simulink model "simpleTankTest"  (R2020b)
settings: Solver=VariableStepAuto  StartTime=0.0  StopTime=50  RelTol=1e-3
libraries: fl_lib x11, nesl_utility x10, SimscapeCustomBlocks_lib x2
settings Model: Creator=Edward  LastModifiedBy=Edward

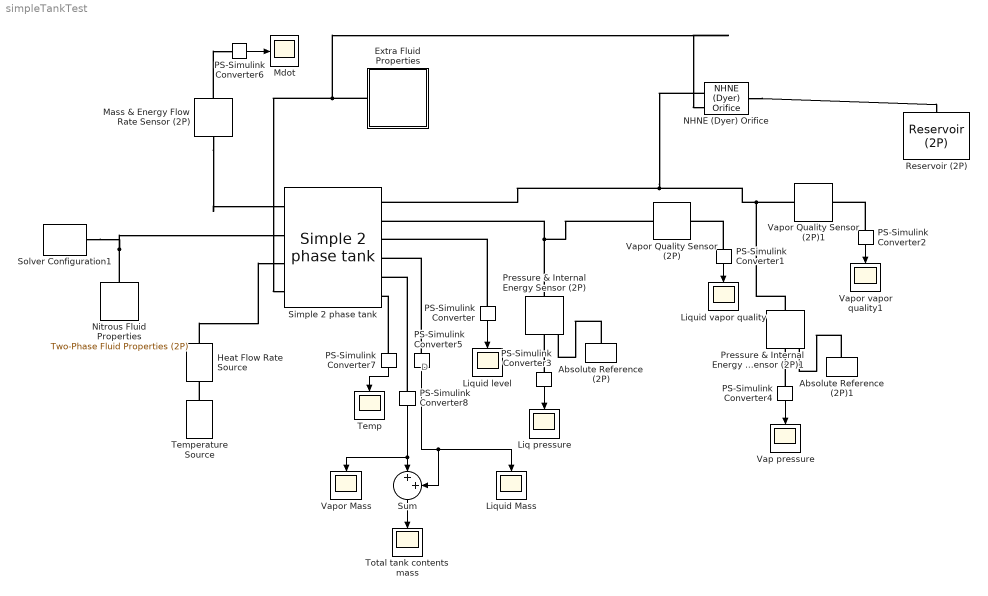
== system simpleTankTest ==
  note: D
  Absolute Reference (2P) : fl_lib/Two-Phase Fluid/Elements/Absolute Reference (2P)
      settings: SourceProductBaseCode=SS
  Absolute Reference (2P)1 : fl_lib/Two-Phase Fluid/Elements/Absolute Reference (2P)
      settings: SourceProductBaseCode=SS
  Extra Fluid Properties : Subsystem  ReferencedSubsystem=nitrousExtraFluidProps
  Heat Flow Rate Source : fl_lib/Thermal/Thermal Sources/Heat Flow Rate Source  heat_flow=900 W
      settings: SourceProductBaseCode=SS  InternalSimscapePortConfiguration="{\"Bottom\":[],\"Left\":[{\"id\":\"B\",\"label\":\"B\",\"type\":\"foundation.thermal.thermal\"}],\"Right\":[{\"id\":\"A\",\"label\":\"A\",\"type\":\"foundation.thermal.thermal\"}],\"Top\":[]}"
  Liq pressure : Scope
  Liquid Mass : Scope
  Liquid level : Scope
  Liquid vapor quality : Scope
  Mass & Energy Flow Rate Sensor (2P) : fl_lib/Two-Phase Fluid/Sensors/Mass & Energy Flow Rate Sensor (2P)
      settings: SourceProductBaseCode=SS  InternalSimscapePortConfiguration="{\"Bottom\":[],\"Left\":[{\"id\":\"A\",\"label\":\"A\",\"type\":\"foundation.two_phase_fluid.two_phase_fluid\"}],\"Right\":[{\"id\":\"B\",\"label\":\"B\",\"type\":\"foundation.two_phase_fluid.two_phase_fluid\"},{\"id\":\"M\",\"label\":\"M\",\"type\":\"output\"},{\"id\":\"PHI\",\"label\":\"Phi\",\"type\":\"output\"}],\"Top\":[]}"
  Mdot : Scope
  NHNE (Dyer) Orifice : SimscapeCustomBlocks_lib/NHNE (Dyer) Orifice  area=0.01 m^2  orifice_area=0.25*pi*(1.5e-3)^2 m^2  Cd=0.8
      settings: InternalSimscapePortConfiguration="{\"Bottom\":[],\"Left\":[{\"id\":\"A\",\"label\":\"A\",\"type\":\"foundation.two_phase_fluid.two_phase_fluid\"}],\"Right\":[{\"id\":\"B\",\"label\":\"B\",\"type\":\"foundation.two_phase_fluid.two_phase_fluid\"}],\"Top\":[{\"id\":\"Props\",\"label\":\"Props\",\"type\":\"SimscapeCustomBlocks.customFluidDomain.extra_two_phase_fluid_props\"}]}"
  Nitrous Fluid Properties : fl_lib/Two-Phase Fluid/Utilities/Two-Phase Fluid Properties (2P)  u_min=Sim.nitrousFluidTable.u_min kJ/kg  u_max=Sim.nitrousFluidTable.u_max kJ/kg  unorm_liq=Sim.nitrousFluidTable.liquid.unorm  unorm_vap=Sim.nitrousFluidTable.vapor.unorm  p_TLU=Sim.nitrousFluidTable.p MPa  v_liq=Sim.nitrousFluidTable.liquid.v m^3/kg  v_vap=Sim.nitrousFluidTable.vapor.v m^3/kg  s_liq=Sim.nitrousFluidTable.liquid.s kJ/kg/K  s_vap=Sim.nitrousFluidTable.vapor.s kJ/kg/K  T_liq=Sim.nitrousFluidTable.liquid.T K  T_vap=Sim.nitrousFluidTable.vapor.T K  nu_liq=Sim.nitrousFluidTable.liquid.nu mm^2/s  nu_vap=Sim.nitrousFluidTable.vapor.nu mm^2/s  k_liq=Sim.nitrousFluidTable.liquid.k W/(m*K)  k_vap=Sim.nitrousFluidTable.vapor.k W/(m*K)  Pr_liq=Sim.nitrousFluidTable.liquid.Pr  Pr_vap=Sim.nitrousFluidTable.vapor.Pr  u_sat_liq=Sim.nitrousFluidTable.liquid.u_sat kJ/kg  u_sat_vap=Sim.nitrousFluidTable.vapor.u_sat kJ/kg  p_crit=Sim.nitrousFluidTable.p_crit MPa  critical_region=foundation.enum.critical_region.clip  p_crit_fraction=0.12  p_atm=0.101325 MPa  q_rev=0.01 Pa
      settings: SourceProductBaseCode=SS  InternalSimscapePortConfiguration="{\"Bottom\":[],\"Left\":[],\"Right\":[{\"id\":\"A\",\"label\":\"\",\"type\":\"foundation.two_phase_fluid.two_phase_fluid\"}],\"Top\":[]}"
  PS-Simulink Converter{,1..8} (9 alike) : nesl_utility/PS-Simulink Converter  PhysicalDomain=network_engine_domain  SubClassName=ps_output  LeftPortType=input  RightPortType=output  PseudoPeriodic=off  Frequencies=[]  Unit=inherit  AffineConversion=off
  Pressure & Internal Energy Sensor (2P) : fl_lib/Two-Phase Fluid/Sensors/Pressure & Internal Energy Sensor (2P)
      settings: SourceProductBaseCode=SS  InternalSimscapePortConfiguration="{\"Bottom\":[],\"Left\":[{\"id\":\"A\",\"label\":\"A\",\"type\":\"foundation.two_phase_fluid.two_phase_fluid\"}],\"Right\":[{\"id\":\"B\",\"label\":\"B\",\"type\":\"foundation.two_phase_fluid.two_phase_fluid\"},{\"id\":\"P\",\"label\":\"P\",\"type\":\"output\"},{\"id\":\"U\",\"label\":\"U\",\"type\":\"output\"}],\"Top\":[]}"
  Pressure & Internal Energy Sensor (2P)1 : fl_lib/Two-Phase Fluid/Sensors/Pressure & Internal Energy Sensor (2P)
      settings: SourceProductBaseCode=SS  InternalSimscapePortConfiguration="{\"Bottom\":[],\"Left\":[{\"id\":\"A\",\"label\":\"A\",\"type\":\"foundation.two_phase_fluid.two_phase_fluid\"}],\"Right\":[{\"id\":\"B\",\"label\":\"B\",\"type\":\"foundation.two_phase_fluid.two_phase_fluid\"},{\"id\":\"P\",\"label\":\"P\",\"type\":\"output\"},{\"id\":\"U\",\"label\":\"U\",\"type\":\"output\"}],\"Top\":[]}"
  Reservoir (2P) : fl_lib/Two-Phase Fluid/Elements/Reservoir (2P)  pressure_spec=foundation.enum.pressure_spec.specified  reservoir_pressure=10 bar  energy_spec=foundation.enum.energy_spec.temperature  reservoir_temperature=293.15 K  reservoir_quality=0.5  reservoir_void_fraction=0.5  reservoir_enthalpy=1500 kJ/kg  reservoir_internal_energy=1500 kJ/kg  area_A=0.01 m^2
      settings: SourceProductBaseCode=SS
  Simple 2 phase tank : SimscapeCustomBlocks_lib/Simple 2 phase tank  areaL=0.01 m^2  areaV=0.01 m^2  tank_volume=Sim.runTank.volume m^3  alpha_L=100 W/(m^2 * K)  alpha_V=20 W/(m^2 * K)  heat_surface_area=2 m^2  p_init=60 bar  liq_vol_frac_init=0.5
      settings: InternalSimscapePortConfiguration="{\"Bottom\":[],\"Left\":[{\"id\":\"AV\",\"label\":\"AV\",\"type\":\"foundation.two_phase_fluid.two_phase_fluid\"},{\"id\":\"AL\",\"label\":\"AL\",\"type\":\"foundation.two_phase_fluid.two_phase_fluid\"},{\"id\":\"H\",\"label\":\"H\",\"type\":\"foundation.thermal.thermal\"}],\"Right\":[{\"id\":\"BV\",\"label\":\"BV\",\"type\":\"foundation.two_phase_fluid.two_phase_fluid\"},{\"id\":\"BL\",\"label\":\"BL\",\"type\":\"foundation.two_phase_fluid.two_phase_fluid\"},{\"id\":\"L\",\"label\":\"L\",\"type\":\"output\"},{\"id\":\"ML\",\"label\":\"ML\",\"type\":\"output\"},{\"id\":\"MV\",\"label\":\"MV\",\"type\":\"output\"},{\"id\":\"T\",\"label\":\"T\",\"type\":\"output\"}],\"Top\":[{\"id\":\"Props\",\"label\":\"Props\",\"type\":\"SimscapeCustomBlocks.customFluidDomain.extra_two_phase_fluid_props\"}]}"
  Solver Configuration1 : nesl_utility/Solver Configuration  PhysicalDomain=network_engine_domain  SubClassName=solver  LeftPortType=input  RightPortType=generic  Tones=[]  Harmonics=[]  SimulateNoise=off  Profile=off  UseLocalSampling=off  EnableSwitchedLinearOptims=on  FrequencyDomain=off  UseCCode=off  RelTol=0.001  AbsTol=1e-06  MinStep=1e-09  ToWorkspace=off  RevertToSquareIcSolve=off  NumHomotopyIterations=100  PhasorMode=off  PhasorModeNumHarmonics=1  DoDC=off  ResidualTolerance=1e-9  UseLocalSolver=off  LocalSolverChoice=NE_BACKWARD_EULER_ADVANCER  LocalSolverSampleTime=0.001  DoFixedCost=off  MaxNonlinIter=3  MaxModeIter=2  ComputeImpulses=off  ImpulseIterations=2  LinearAlgebra=auto  EquationFormulation=NE_TIME_EF  DelaysMemoryBudget=1024  AutomaticFiltering=on  FilteringTimeConstant=0.001  PartitionStorageMethod=AS_NEEDED  PartitionMemoryBudget=1024  PartitionMethod=ROBUST
  Sum : Sum  Inputs=|++
  Temp : Scope
  Temperature Source : fl_lib/Thermal/Thermal Sources/Temperature Source  temperature=293.15 K
  Total tank contents mass : Scope
  Vap pressure : Scope
  Vapor Mass : Scope
  Vapor Quality Sensor (2P) : fl_lib/Two-Phase Fluid/Sensors/Vapor Quality Sensor (2P)  vapor_fraction_spec=foundation.enum.vapor_fraction_spec.quality
      settings: SourceProductBaseCode=SS  InternalSimscapePortConfiguration="{\"Bottom\":[],\"Left\":[{\"id\":\"A\",\"label\":\"A\",\"type\":\"foundation.two_phase_fluid.two_phase_fluid\"}],\"Right\":[{\"id\":\"X\",\"label\":\"X\",\"type\":\"output\"}],\"Top\":[]}"
  Vapor Quality Sensor (2P)1 : fl_lib/Two-Phase Fluid/Sensors/Vapor Quality Sensor (2P)  vapor_fraction_spec=foundation.enum.vapor_fraction_spec.quality
      settings: SourceProductBaseCode=SS  InternalSimscapePortConfiguration="{\"Bottom\":[],\"Left\":[{\"id\":\"A\",\"label\":\"A\",\"type\":\"foundation.two_phase_fluid.two_phase_fluid\"}],\"Right\":[{\"id\":\"X\",\"label\":\"X\",\"type\":\"output\"}],\"Top\":[]}"
  Vapor vapor quality1 : Scope
  wires:
  PS-Simulink Converter/1 -> Liquid level/1
  PS-Simulink Converter1/1 -> Liquid vapor quality/1
  PS-Simulink Converter2/1 -> Vapor vapor quality1/1
  PS-Simulink Converter3/1 -> Liq pressure/1
  PS-Simulink Converter4/1 -> Vap pressure/1
  PS-Simulink Converter5/1 -> Sum/2, Liquid Mass/1
  PS-Simulink Converter6/1 -> Mdot/1
  PS-Simulink Converter7/1 -> Temp/1
  PS-Simulink Converter8/1 -> Sum/1, Vapor Mass/1
  Sum/1 -> Total tank contents mass/1
  connections:
  Nitrous Fluid Properties/RConn1 -- Solver Configuration1/RConn1 -- Simple 2 phase tank/LConn2
  PS-Simulink Converter/LConn1 -- Simple 2 phase tank/RConn3
  Vapor Quality Sensor (2P)/LConn1 -- Simple 2 phase tank/RConn2 -- Pressure & Internal Energy Sensor (2P)/LConn1
  PS-Simulink Converter1/LConn1 -- Vapor Quality Sensor (2P)/RConn1
  PS-Simulink Converter2/LConn1 -- Vapor Quality Sensor (2P)1/RConn1
  Vapor Quality Sensor (2P)1/LConn1 -- Pressure & Internal Energy Sensor (2P)1/LConn1 -- Simple 2 phase tank/RConn1 -- NHNE (Dyer) Orifice/LConn1
  Absolute Reference (2P)/LConn1 -- Pressure & Internal Energy Sensor (2P)/RConn1
  PS-Simulink Converter3/LConn1 -- Pressure & Internal Energy Sensor (2P)/RConn2
  PS-Simulink Converter4/LConn1 -- Pressure & Internal Energy Sensor (2P)1/RConn2
  Absolute Reference (2P)1/LConn1 -- Pressure & Internal Energy Sensor (2P)1/RConn1
  PS-Simulink Converter5/LConn1 -- Simple 2 phase tank/RConn4
  Mass & Energy Flow Rate Sensor (2P)/LConn1 -- Simple 2 phase tank/LConn1
  Mass & Energy Flow Rate Sensor (2P)/RConn2 -- PS-Simulink Converter6/LConn1
  Extra Fluid Properties/RConn1 -- Simple 2 phase tank/LConn4 -- NHNE (Dyer) Orifice/LConn2
  PS-Simulink Converter8/LConn1 -- Simple 2 phase tank/RConn5
  NHNE (Dyer) Orifice/RConn1 -- Reservoir (2P)/LConn1
  Temperature Source/LConn1 -- Heat Flow Rate Source/RConn1
  Heat Flow Rate Source/LConn1 -- Simple 2 phase tank/LConn3
  PS-Simulink Converter7/LConn1 -- Simple 2 phase tank/RConn6
